simulink model "comparacao_linear_e_nao"  (R2023b)
settings: Solver=VariableStepAuto  StartTime=0.0  StopTime=25  RelTol=1e-3
settings Model: Creator=luang  LastModifiedBy=Geovanne
settings SolverCC: AlgebraicLoopSolver=TrustRegion
settings DebuggingCC: UnconnectedInputMsg=warning  UnconnectedOutputMsg=warning  UnconnectedLineMsg=warning
settings ModelReferenceCC: EnableRefExpFcnMdlSchedulingChecks=on

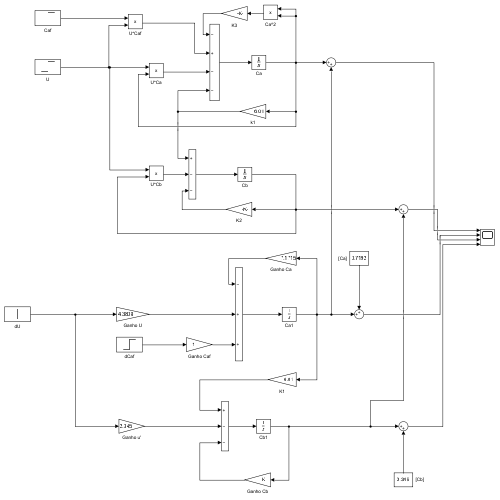
[thumbnail: Simulink's stored preview of the top-level diagram]
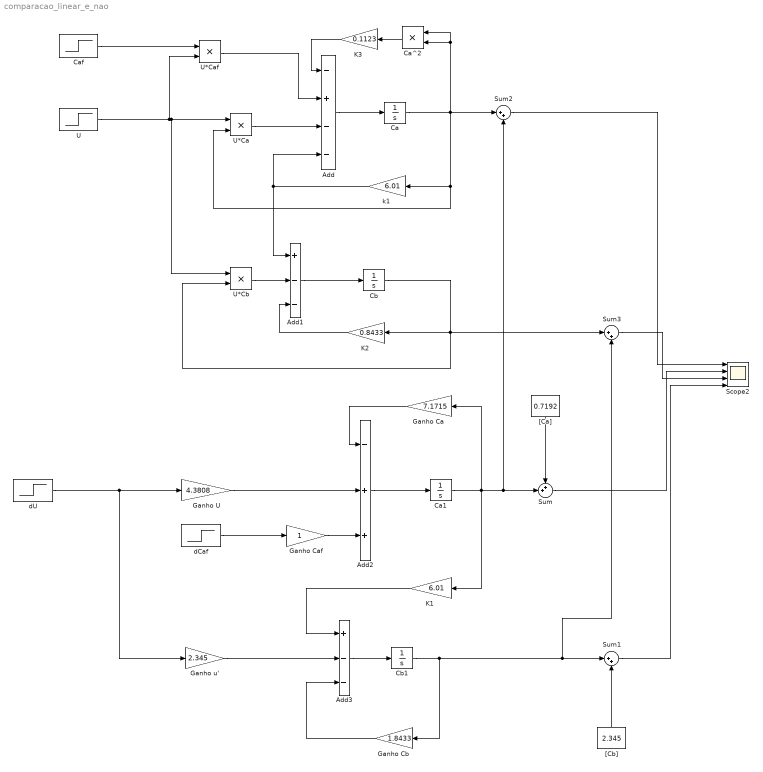
== system comparacao_linear_e_nao ==
  Add : Sum  Inputs=-+--
  Add1 : Sum  Inputs=+--
  Add2 : Sum  Inputs=-++
  Add3 : Sum  Inputs=+--
  Ca : Integrator
  Ca1 : Integrator
  Ca^2 : Product
  Caf : Step  Time=0  After=5.1  SampleTime=0
  Cb : Integrator
  Cb1 : Integrator
  Ganho Ca : Gain  Gain=7.1715
  Ganho Caf : Gain
  Ganho Cb : Gain  Gain=1.8433
  Ganho U : Gain  Gain=4.3808
  Ganho u' : Gain  Gain=2.345
  K1 : Gain  Gain=6.01
  K2 : Gain  Gain=0.8433
  K3 : Gain  Gain=0.1123
  Scope2 : Scope  NumInputPorts=4
  Sum : Sum  Inputs=++|
  Sum1 : Sum  Inputs=|++
  Sum2 : Sum  Inputs=|++
  Sum3 : Sum  Inputs=|++
  U : Step  Time=0  SampleTime=0
  U*Ca : Product
  U*Caf : Product
  U*Cb : Product
  "[Ca]" : Constant  Value=0.7192
  "[Cb]" : Constant  Value=2.345
  dCaf : Step  Time=15  After=0.1  SampleTime=0
  dU : Step  Time=15  After=0.1  SampleTime=0
  k1 : Gain  Gain=6.01
  wires:
  k1/1 -> Add1/1, Add/4
  U*Cb/1 -> Add1/2
  K2/1 -> Add1/3
  Add1/1 -> Cb/1
  Ca/1 -> Sum2/1, Ca^2/2, Ca^2/1, k1/1, U*Ca/2
  U*Ca/1 -> Add/3
  Ca^2/1 -> K3/1
  Add/1 -> Ca/1
  K3/1 -> Add/1
  Cb/1 -> U*Cb/2, Sum3/1, K2/1
  U*Caf/1 -> Add/2
  "[Ca]"/1 -> Sum/1
  "[Cb]"/1 -> Sum1/2
  Ganho Cb/1 -> Add3/3
  dU/1 -> Ganho u'/1, Ganho U/1
  Add2/1 -> Ca1/1
  Ganho Ca/1 -> Add2/1
  K1/1 -> Add3/1
  dCaf/1 -> Ganho Caf/1
  Ca1/1 -> Ganho Ca/1, K1/1, Sum/2, Sum2/2
  Ganho u'/1 -> Add3/2
  Add3/1 -> Cb1/1
  Cb1/1 -> Ganho Cb/1, Sum1/1, Sum3/2
  Sum/1 -> Scope2/2
  Sum1/1 -> Scope2/4
  Ganho U/1 -> Add2/2
  Ganho Caf/1 -> Add2/3
  Sum2/1 -> Scope2/1
  Sum3/1 -> Scope2/3
  Caf/1 -> U*Caf/1
  U/1 -> U*Cb/1, U*Ca/1, U*Caf/2
